simulink model "transferfunction9A_harness_with_control_loop"  (R2022b)
settings: Solver=VariableStepAuto  StartTime=time_in(1)  StopTime=time_in(end)  RelTol=1e-3
values from neighbouring files (symbols this model uses):
  Kc = 0.25    [transferfunction9_Kobe_Michiels.m]
  tau_d = Td/(10*Kc)    (= 0.004)    [transferfunction9_Kobe_Michiels.m]
  Td = 0.01    [transferfunction9_Kobe_Michiels.m]
  Ti = 0.01    [transferfunction9_Kobe_Michiels.m]
  time_delay = 0.02    [transferfunction9_Kobe_Michiels.m]
settings Model: Creator=Kobe Michiels  LastModifiedBy=Kobe Michiels
settings DataIOCC: ExternalInput=[time_in, input]  LoadExternalInput=on  SaveFormat=Array  SignalLogging=off  DSMLogging=off  TimeSaveName=time_out  OutputSaveName=response
settings DebuggingCC: AlgebraicLoopMsg=none

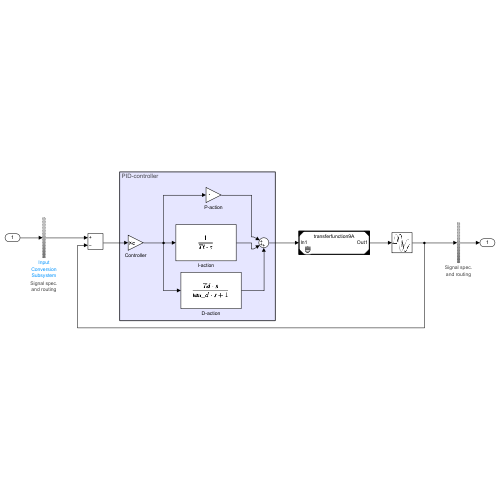
[thumbnail: Simulink's stored preview of the top-level diagram]
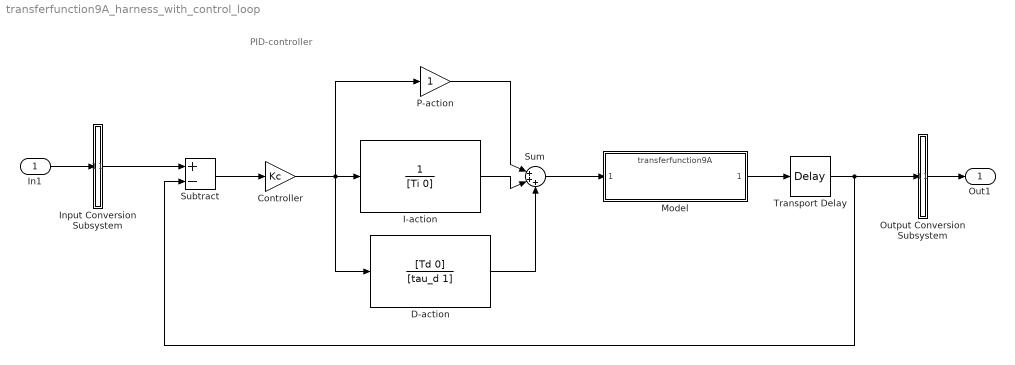
== system transferfunction9A_harness_with_control_loop ==
  note: PID-controller
  In1 : Inport  OutDataTypeStr=double  PortDimensions=[1]  SampleTime=0
  Controller : Gain  Gain=Kc
  D-action : TransferFcn  Numerator=[Td 0]  Denominator=[tau_d 1]  ParameterTunability=Unconstrained
  I-action : TransferFcn  Denominator=[Ti 0]  ParameterTunability=Unconstrained
  Input Conversion Subsystem : Subsystem  Tag=__SLT_ICS__  Description=|
      | Signal spec.
      | and routing
      settings: AttributesFormatString=%<Description>
  Model : ModelReference  ModelNameDialog=transferfunction9A.slxp  ModelReferenceVersion=1.38  CopyOfModelProtected=on
  Output Conversion Subsystem : Subsystem  Tag=__SLT_OCS__  Description=|
      | Signal spec.
      | and routing
      settings: AttributesFormatString=%<Description>
  P-action : Gain
  Subtract : Sum  Inputs=+-
  Sum : Sum  Inputs=|+++
  Transport Delay : TransportDelay  DelayTime=time_delay
  Out1 : Outport
  wires:
  Model/1 -> Transport Delay/1
  Input Conversion Subsystem/1(Outport_1) -> Subtract/1
  In1/1 -> Input Conversion Subsystem/1(Inport_1)
  Output Conversion Subsystem/1(Outport_1) -> Out1/1
  Transport Delay/1 -> Output Conversion Subsystem/1(Inport_1), Subtract/2
  Sum/1 -> Model/1
  Subtract/1 -> Controller/1
  P-action/1 -> Sum/1
  D-action/1 -> Sum/3
  Controller/1 -> D-action/1, I-action/1, P-action/1
  I-action/1 -> Sum/2

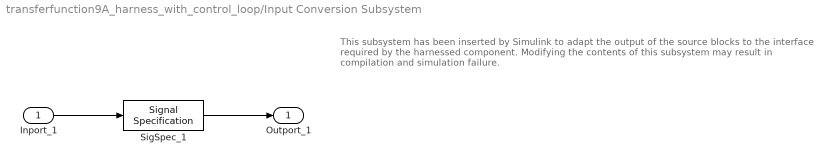
== system transferfunction9A_harness_with_control_loop/Input Conversion Subsystem ==
  note: This subsystem has been inserted by Simulink to adapt the output of the source blocks to the interface required by the harnessed component.
      |  Modifying the contents of this subsystem may result in compilation and simulation failure.
  Inport_1 : Inport
  SigSpec_1 : SignalSpecification  OutDataTypeStr=double  Dimensions=[1]  SampleTime=[0, 0]
  Outport_1 : Outport
  wires:
  SigSpec_1/1 -> Outport_1/1
  Inport_1/1 -> SigSpec_1/1

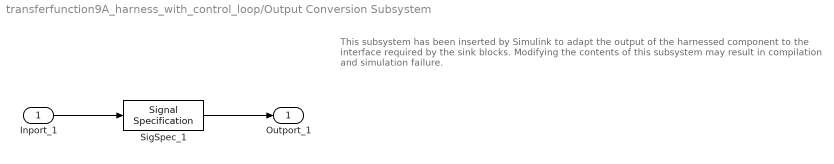
== system transferfunction9A_harness_with_control_loop/Output Conversion Subsystem ==
  note: This subsystem has been inserted by Simulink to adapt the output of the harnessed component to the interface required by the sink blocks.
      |  Modifying the contents of this subsystem may result in compilation and simulation failure.
  Inport_1 : Inport
  SigSpec_1 : SignalSpecification  OutDataTypeStr=double  Dimensions=[1]
  Outport_1 : Outport
  wires:
  Inport_1/1 -> SigSpec_1/1
  SigSpec_1/1 -> Outport_1/1
